simulink model "RefModel_Task"  (R2020a)
(part 4 of 5)

    |         isAutoMode_globalvar && ...
    |         PathModeOut.whereIsUAV == ENUM_Where.InTheAir && ...
    |         ComFlightOut.curLLA(3) < CmdParam_altitude - 22
    |     duration = duration + Ts;
    |     if duration > 0.3
    |         flag = true;
    |     end
    | end
  function flag = isHeightTooLow_HoverDown:
    | function flag = isHeightTooLow_HoverDown
    | % 在盘旋下降模式判断高度过低
    | persistent duration
    | if isempty(duration)
    |     duration = 0;
    | end
    | modeCond = PathModeOut.flightTaskMode == ENUM_FlightTaskMode.HoverDownMode;
    | flag = false;
    | if modeCond && ...
    |         IN_SignalIntegrity.SensorStatus.radar1 == ENUM_SensorHealthStatus.Health && ...
    |         IN_SENSOR.radar1.Range < TaskParam.minHeightInFix && IN_SENSOR.radar1.Range ~=0 &&...
    |         isUavInFix && ...
    |         isAutoMode_globalvar && ...
    |         PathModeOut.whereIsUAV == ENUM_Where.InTheAir
    |     duration = duration + Ts;
    |     if duration > 1
    |         flag = true;
    |         if ComFlightOut.curLLA(3) > CmdParam_altitude % 当前高度大于切换高度时,将当前高度改为切换高度
    |             CmdParam_altitude = ComFlightOut.curLLA(3);
    |             PathModeOut.heightCmd = CmdParam_altitude;
    |         else % 当前高度小于切换高度时, 仍使用原切换高度
    |             
    |         end
    |     end
    | end
  function initWindParam:
    | function initWindParam
    | WindParamOut.sailWindSpeed = 0;
    | WindParamOut.sailWindHeading = 0;
    | WindParamOut.windSpeedMax = 0;
    | WindParamOut.windSpeedMin = 0;
    | WindParamOut.maxWindHeading = 0;
  function flag = isAnyGPSOk:
    | function flag = isAnyGPSOk
    | flag = false;
    | if IN_SignalIntegrity.SensorStatus.ublox1 == ENUM_SensorHealthStatus.Health || ...
    |         IN_SignalIntegrity.SensorStatus.ublox1 == ENUM_SensorHealthStatus.Degrade || ...
    |         IN_SignalIntegrity.SensorStatus.um482 == ENUM_SensorHealthStatus.Degrade || ...
    |          IN_SignalIntegrity.SensorStatus.um482 == ENUM_SensorHealthStatus.Health
    |     flag = true;
    | end
  function flag = canContinueFly:
    | function flag = canContinueFly
    | persistent duration
    | if isempty(duration)
    |     duration = 0;
    | end
    | flag = true;
    | % if IN_SignalIntegrity.SystemHealthStatus ~= ENUM_SystemHealthStatus.SystemHealth && ... % 传感器系统不正常
    | %         IN_SignalIntegrity.SystemHealthStatus ~= ENUM_SystemHealthStatus.DontTakeOff && ...
    | %         IN_SignalIntegrity.SystemHealthStatus ~= ENUM_SystemHealthStatus.NeedToReturn
    | if IN_SignalIntegrity.SystemHealthStatus == ENUM_SystemHealthStatus.CanNotFly % 传感器系统 CanNotFly
    |     duration = duration + Ts;
    |     if duration > 10 && isUavInRotor% 大于一定时间后进行判定
    |         flag = false;
    |     end
    |     if duration > 15 && isUavInFix% 大于一定时间后进行判定
    |         flag = false;
    |     end    
    | else
    |     duration = 0;
    | end
  function flag = isNeedToReturn:
    | function flag = isNeedToReturn
    | persistent duration
    | if isempty(duration)
    |     duration = 0;
    | end
    | flag = false;
    | if IN_SignalIntegrity.SystemHealthStatus == ENUM_SystemHealthStatus.NeedToReturn
    |     duration = duration + Ts;
    |     if duration > 10
    |         flag = true;
    |     end
    | else
    |     duration = 0;
    | end
    | 
    | % function flag = isSensorSystemHealth
    | % flag = true;
    | % if IN_SignalIntegrity.SystemHealthStatus ~= ENUM_SystemHealthStatus.SystemHealth && ... % 传感器不正常
    | %         IN_SignalIntegrity.SystemHealthStatus ~= ENUM_SystemHealthStatus.DontTakeOff
    | %     flag = false;
    | % end
  function updateFenseDist:
    | function updateFenseDist
    | if TaskParam.enableFenseDistUpdate
    |     if RTInfo.maxDist_Path2Home > fenseValidDist
    |         fenseValidDist = RTInfo.maxDist_Path2Home + 1000;
    |         fprintf('Fastest path point is farther than preset fensedist, update fensedist to %.0f!\n',fenseValidDist);
    |     end
    |     if fenseValidDist > FlightPerfParam.maxFixWingRange/2
    |         fprintf('Fensedist is father than half of uav max range which is %.0f!\n',FlightPerfParam.maxFixWingRange/2);
    |     end    
    | end
    | RTInfo.realtimeFenseDist = fenseValidDist;
  function flag_out  = isLargeAttitudeLong_Fix(pitch_in, threshold_pitch):
    | function flag_out  = isLargeAttitudeLong_Fix(pitch_in, threshold_pitch)
    | persistent du period pitchFlagSet 
    | nFlag = 6;
    | if isempty(du)
    |     du = 0; 
    |     period = 0;
    |     pitchFlagSet = zeros(nFlag,1);
    | end
    | period = period + Ts;
    | % threshold_pitch = 35*pi/180;
    | value_period = 3; % sec
    | if period >= value_period
    |     period = 0;
    |     pitchFlagSet(1:end-1) = pitchFlagSet(2:end);
    |     pitchFlagSet(end) = 0;
    | else
    |     % 在周期内，更新flag值
    |     if abs(pitch_in) > threshold_pitch
    |         pitchFlagSet(end) = 1;
    |     end
    | end
    | % if PathModeOut.flightTaskMode == ENUM_FlightTaskMode.GroundStandByMode 
    | 
    | %%
    | flag_out = false;
    | if sum(pitchFlagSet) >= 2 || abs(pitch_in) > 1.3*threshold_pitch
    |     printDebugInfo('AirspeedFault_Protect','LargePitch Fix')
    | %     RTInfo.Task = ENUM_RTInfo_Task.TaskLog_Protect_Airspeed_LargePitch; % 更新RT信息
    | %     updateLogDataBuffer(ENUM_TaskLogBlockName.TASKLOG_FlightMode,RTInfo.Task,'write'); % 更新log缓存    
    |     flag_out = true;
    | else
    |     flag_out = false;
    | end
  function flag_out  = isLargeAttitudeLong_Fix_Level(pitch_in, threshold_pitch):
    | function flag_out  = isLargeAttitudeLong_Fix_Level(pitch_in, threshold_pitch)
    | persistent du period pitchFlagSet 
    | nFlag = 6;
    | if isempty(du)
    |     du = 0; 
    |     period = 0;
    |     pitchFlagSet = zeros(nFlag,1);
    | end
    | period = period + Ts;
    | % threshold_pitch = 35*pi/180;
    | value_period = 3; % sec
    | if period >= value_period
    |     period = 0;
    |     pitchFlagSet(1:end-1) = pitchFlagSet(2:end);
    |     pitchFlagSet(end) = 0;
    | else
    |     % 在周期内，更新flag值
    |     if abs(pitch_in) > threshold_pitch
    |         pitchFlagSet(end) = 1;
    |     end
    | end
    | % if PathModeOut.flightTaskMode == ENUM_FlightTaskMode.GroundStandByMode 
    | 
    | %%
    | flag_out = false;
    | if sum(pitchFlagSet) >= 2 || abs(pitch_in) > 1.3*threshold_pitch
    |     printDebugInfo('AirspeedFault_Protect','LargePitch Fix Level')
    | %     RTInfo.Task = ENUM_RTInfo_Task.TaskLog_Protect_Airspeed_LargePitch; % 更新RT信息
    | %     updateLogDataBuffer(ENUM_TaskLogBlockName.TASKLOG_FlightMode,RTInfo.Task,'write'); % 更新log缓存    
    |     flag_out = true;
    | else
    |     flag_out = false;
    | end
  function flag_out  = isVdTooHigh(Vd_in):
    | function flag_out  = isVdTooHigh(Vd_in)
    | persistent pVd du
    | if isempty(pVd)
    |     du = 0;
    |     pVd = Vd_in;
    | end
    | threshold_Vd = 8;
    | if abs(Vd_in) > threshold_Vd
    |     du = du + Ts; % sec
    | else
    |     du = 0;
    | end
    | if du > 1 % 大于阈值 1 sec
    |     printDebugInfo('AirspeedFault_Protect','LargeVd')
    |     RTInfo.Task = ENUM_RTInfo_Task.TaskLog_Protect_Airspeed_LargeVd; % 更新RT信息
    |     updateLogDataBuffer(ENUM_TaskLogBlockName.TASKLOG_FlightMode,RTInfo.Task,'write'); % 更新log缓存         
    |     flag_out = true;
    | else
    |     flag_out = false;
    | end
  function flag  = isAngularVelOrAccTooHighInFix:
    | function flag  = isAngularVelOrAccTooHighInFix
    | persistent pWx pWy pWz pAz du_wx du_wy du_wz du_az
    | wx = IN_SENSOR.IMU1.gyro_x;
    | wy = IN_SENSOR.IMU1.gyro_y;
    | wz = IN_SENSOR.IMU1.gyro_z;
    | az = IN_SENSOR.IMU1.accel_z;
    | if isempty(pWx)
    |     du = 0;
    |     pWx = wx;
    |     pWy = wy;
    |     pWz = wz;
    |     pAz = az;
    |     du_wx = 0;
    |     du_wy = 0;
    |     du_wz = 0;
    |     du_az = 0;
    | end
    | kW = 0.9;
    | pWx = kW*pWx+(1-kW)*wx;
    | pWy = kW*pWy+(1-kW)*wy;
    | pWz = kW*pWz+(1-kW)*wz;
    | pAz = kW*pAz+(1-kW)*az;
    | threshold_w = 2; % rad/s
    | threshold_az = 22; % m/s^2
    | %%
    | if abs(pWx) > threshold_w
    |     du_wx =  du_wx + Ts;
    | else
    |     du_wx = 0;
    | end
    | if abs(pWy) > threshold_w
    |     du_wy =  du_wy + Ts;
    | else
    |     du_wy = 0;
    | end
    | if abs(pWz) > threshold_w
    |     du_wz =  du_wz + Ts;
    | else
    |     du_wz = 0;
    | end
    | if abs(pAz) > threshold_az
    |     du_az =  du_az + Ts;
    | else
    |     du_az = 0;
    | end
    | %%
    | flag = false;
    | if du_wx > 3 || du_wy > 3 || du_wz > 3 || du_az > 3
    |     flag = true;
    | end
    | %% 
    | if ~isUavInFix
    |     flag = false;
    | end
    | %%
    | if flag
    |     printDebugInfo('AirspeedFault_Protect','LargeAngularVelOrAccz')
    |     RTInfo.Task = ENUM_RTInfo_Task.TaskLog_Protect_Airspeed_LargeAngularVelOrAccz; % 更新RT信息
    |     updateLogDataBuffer(ENUM_TaskLogBlockName.TASKLOG_FlightMode,RTInfo.Task,'write'); % 更新log缓存        
    | end
  function flag  = isNeedToRotor:
    | function flag  = isNeedToRotor
    | flag = false;
    | if (isAngularVelOrAccTooHighInFix || isVdTooHigh(ComFlightOut.curVelNED(3))) && ...
    |         isUavInFix
    |     flag = true;
    | end
  function flag  = isNeedToGoHome:
    | function flag  = isNeedToGoHome
    | flag = false;
    | if isUavInFix
    |     % 针对所有固定翼模式
    |     if isLargeAttitudeLong_Fix(ComFlightOut.curEuler(2),35*pi/180)
    |         flag = true;
    |     end
    |     if isCurrentHigh_Fix(abs(IN_MAV.mavlink_msg_mission_current(1).current),1.5*TaskParam.levelFixcurrentThreshold)
    | %         flag = true;
    |     end
    |     % 针对平飞模式（航线模式 返航模式）
    |     if (PathModeOut.flightTaskMode == ENUM_FlightTaskMode.GoHomeMode || ...
    |             PathModeOut.flightTaskMode == ENUM_FlightTaskMode.PathFollowMode)
    |         if isLargeAttitudeLong_Fix_Level(ComFlightOut.curEuler(2),20*pi/180)
    |             flag = true;
    |         end
    |         if isCurrentHigh_Fix_Level(abs(IN_MAV.mavlink_msg_mission_current(1).current),TaskParam.levelFixcurrentThreshold)
    |             flag = true;
    |         end
    |     end
    | end
  function flag  = isAllowToToRotor:
    | function flag  = isAllowToToRotor
    | flag = false;
    | distFromHome = distOfTwoLL(ComFlightOut.curHomeLLA(1:2),ComFlightOut.curLLA(1:2));
    | if distFromHome < 500 && ComFlightOut.curLLA(3) < 300 % 离home点近的时候
    |     flag = true;
    | end
  function flag_out  = isCurrentHigh_Fix_Level(current_in, threshold_current):
    | function flag_out  = isCurrentHigh_Fix_Level(current_in, threshold_current)
    | % 固定翼平飞时电流过高（可能是空速管堵，使得实际空速偏小造成姿态、高度波动造成的）
    | flag_out = false;
    | if current_in > threshold_current
    |     flag_out = true;
    | end
  function flag_out  = isCurrentHigh_Fix(current_in, threshold_current):
    | function flag_out  = isCurrentHigh_Fix(current_in, threshold_current)
    | % 固定翼时电流过高（可能是空速管堵，使得实际空速偏小造成姿态、高度波动造成的）
    | flag_out = false;
    | if current_in > threshold_current
    |     flag_out = true;
    | end
  function flag = isVeryHighWind:
    | function flag = isVeryHighWind
    | persistent duration
    | if isempty(duration)
    |     duration = 0;
    | end
    | flag = false;
    | if IN_WindNED.windSpeed_ms > TaskParam.windSpeed_WindSafe &&...% 速度条件
    |         PathModeOut.flightTaskMode ~= ENUM_FlightTaskMode.Rotor2Fix_Mode && ...
    |         PathModeOut.flightTaskMode ~= ENUM_FlightTaskMode.Fix2Rotor_Mode
    |     duration = duration + Ts;
    |     if duration > 2
    |         flag = true;
    |     end
    | else
    |     duration = 0;
    | end
  function flag = eventEnable_UnexpectedToGoHome:
    | function flag = eventEnable_UnexpectedToGoHome
    | flag = true;
    | if PathModeOut.flightTaskMode == ENUM_FlightTaskMode.GoHomeMode || ...
    |     PathModeOut.flightTaskMode == ENUM_FlightTaskMode.LandMode || ...% && double(IN_NAVI.lla(3)) < 20
    |         PathModeOut.flightTaskMode == ENUM_FlightTaskMode.HoverDownMode || ...
    |         (PathModeOut.flightTaskMode == ENUM_FlightTaskMode.Fix2Rotor_Mode && PathModeOut.typeAutoMode == ENUM_AutoModeType.AutoProfile)
    |     flag = false;
    | end
  function flag = eventEnable_UnexpectedToLand:
    | function flag = eventEnable_UnexpectedToLand
    | % 针对所有应急降落流程
    | flag = true;
    | if PathModeOut.flightTaskMode == ENUM_FlightTaskMode.LandMode || ... && double(IN_NAVI.lla(3)) < 15
    |         PathModeOut.flightTaskMode == ENUM_FlightTaskMode.HoverDownMode || ...
    |         PathModeOut.flightTaskMode == ENUM_FlightTaskMode.Fix2Rotor_Mode
    |     flag = false;
    | end
  function flag = isSingleModeRun:
    | function flag = isSingleModeRun
    | flag = false;
    | if PathModeOut.typeAutoMode == ENUM_AutoModeType.SingleModeRun
    |     flag = true;
    | end
  function flag = isBatteryRunOut:
    | function flag = isBatteryRunOut
    | flag = false;
    | %% 条件1：电池电量低于阈值
    | nBattery = length(IN_MAV.mavlink_msg_mission_current);
    | for i = 1:nBattery
    |     if IN_MAV.mavlink_msg_mission_current(i).remaining <= TaskParam.runout_battery_alarm_set
    |         % 如果任意一个电池电量低于预设值
    |         flag = true;
    |         break
    |     end
    | end
  function flag = isLandUncondition:
    | function flag = isLandUncondition
    | flag = false;
    | if isBatteryRunOut
    |     flag = true;
    | end
